simulink model "chapter2"  (R2022a)
settings: Solver=FixedStepAuto  StartTime=0.0  StopTime=1  FixedStep=1e-3  RelTol=1e-3
model workspace (MAT data in the model file):
  a = 0
values from neighbouring files (symbols this model uses):
  A = 10    [Figure2_3.m]    (also in Figure2_9and2_10and2_11.m = A_set(N1-5); parameterLoadForchapter2_4.m = 0.0001; parameterLoadForchapter2_5.m = 0.0001; parameter_load3.m = 0.01)
  Ln = Lns(i)    [Figure2_12and2_13.m]    (also in Figure2_14and2_15.m; Figure2_16and2_17.m; Mchapter2_4.m = LNs(i); parameterLoadForchapter2_5.m = 0.02)
  r = 0.42    [parameterLoadForchapter2_4.m]    (also in parameterLoadForchapter2_5.m; parameter_load3.m)
  v = 100/3.6    (= 27.7777777778)    [Figure2_18_and2_19.m]    (also in Figure2_20_and2_21.m; parameterLoadForchapter2_4.m = 13.8888888889; parameterLoadForchapter2_5.m; parameter_load3.m)
undefined symbols (not defined in the file or in its folder): C1, K1, M1
settings Model: Creator=Spicydel  LastModifiedBy=Spicydel

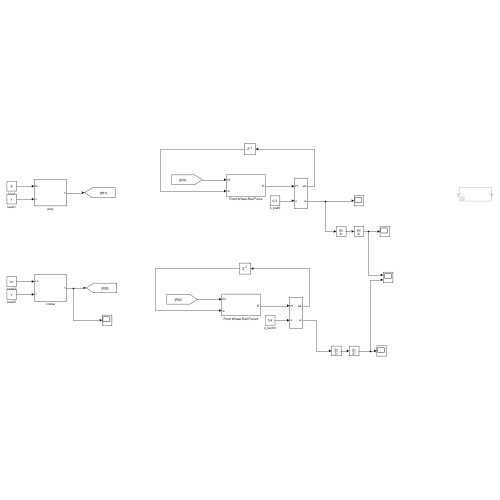
[thumbnail: Simulink's stored preview of the top-level diagram]
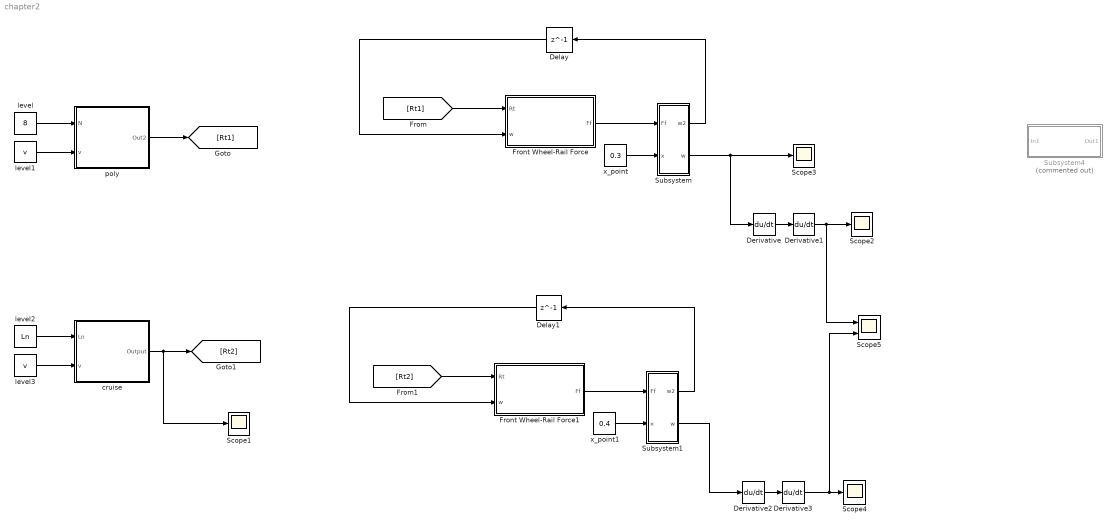
== system chapter2 ==
  Delay : Delay  DelayLength=1
  Delay1 : Delay  DelayLength=1
  Derivative{,1..3} (4 alike) : Derivative
  Front Wheel-Rail Force : Subsystem
  Front Wheel-Rail Force1 : Subsystem
  Scope{1..4} (4 alike) : Scope
  Scope5 : Scope  NumInputPorts=2
  Subsystem : Subsystem
  Subsystem1 : Subsystem
  Subsystem4 : Subsystem  Commented=on
  cruise : Subsystem
  level : Constant  Value=8
  level1 : Constant  Value=v
  level2 : Constant  Value=Ln
  level3 : Constant  Value=v
  poly : Subsystem
  x_point : Constant  Value=0.3
  x_point1 : Constant  Value=0.4
  wires:
  Front Wheel-Rail Force/1(Ff) -> Subsystem/1(Ff)
  x_point/1 -> Subsystem/2(x)
  Derivative/1 -> Derivative1/1
  Delay/1 -> Front Wheel-Rail Force/2(w)
  level/1 -> poly/1(N)
  level1/1 -> poly/2(v)
  poly/1(Out2) -> [Rt1]
  [Rt1] -> Front Wheel-Rail Force/1(Rt)
  cruise/1(Output) -> Scope1/1, [Rt2]
  level3/1 -> cruise/2(v)
  level2/1 -> cruise/1(Ln)
  [Rt2] -> Front Wheel-Rail Force1/1(Rt)
  Delay1/1 -> Front Wheel-Rail Force1/2(w)
  Derivative2/1 -> Derivative3/1
  x_point1/1 -> Subsystem1/2(x)
  Front Wheel-Rail Force1/1(Ff) -> Subsystem1/1(Ff)
  Derivative1/1 -> Scope5/1, Scope2/1
  Derivative3/1 -> Scope5/2, Scope4/1
  Subsystem/1(w2) -> Delay/1
  Subsystem/2(w) -> Derivative/1, Scope3/1
  Subsystem1/1(w2) -> Delay1/1
  Subsystem1/2(w) -> Derivative2/1

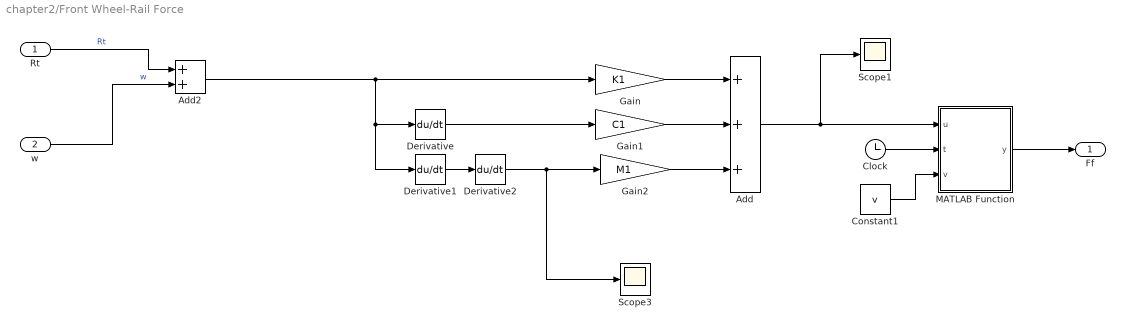
== system chapter2/Front Wheel-Rail Force ==
  Rt : Inport
  w : Inport  Port=2
  Add : Sum  Inputs=+++
  Add2 : Sum
  Clock : Clock
  Constant1 : Constant  Value=v
  Derivative : Derivative
  Derivative1 : Derivative
  Derivative2 : Derivative
  Gain : Gain  Gain=K1
  Gain1 : Gain  Gain=C1
  Gain2 : Gain  Gain=M1
  MATLAB Function : MATLAB Function  TreatAsAtomicUnit=on
  Scope1 : Scope
  Scope3 : Scope
  Ff : Outport
  wires:
  Add2/1 -> Gain/1, Derivative1/1, Derivative/1
  Derivative1/1 -> Derivative2/1
  Gain2/1 -> Add/3
  Gain/1 -> Add/1
  Add/1 -> Scope1/1, MATLAB Function/1(u)
  Rt/1 -> Add2/1  "Rt"
  w/1 -> Add2/2  "w"
  MATLAB Function/1(y) -> Ff/1
  Clock/1 -> MATLAB Function/2(t)
  Constant1/1 -> MATLAB Function/3(v)
  Derivative2/1 -> Scope3/1, Gain2/1
  Derivative/1 -> Gain1/1
  Gain1/1 -> Add/2

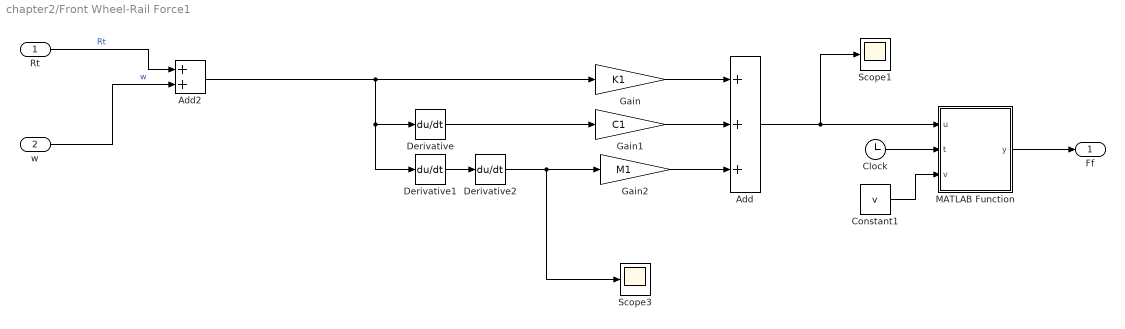
== system chapter2/Front Wheel-Rail Force1 ==
  Rt : Inport
  w : Inport  Port=2
  Add : Sum  Inputs=+++
  Add2 : Sum
  Clock : Clock
  Constant1 : Constant  Value=v
  Derivative : Derivative
  Derivative1 : Derivative
  Derivative2 : Derivative
  Gain : Gain  Gain=K1
  Gain1 : Gain  Gain=C1
  Gain2 : Gain  Gain=M1
  MATLAB Function : MATLAB Function  TreatAsAtomicUnit=on
  Scope1 : Scope
  Scope3 : Scope
  Ff : Outport
  wires:
  Gain1/1 -> Add/2
  Derivative/1 -> Gain1/1
  Derivative2/1 -> Gain2/1, Scope3/1
  Constant1/1 -> MATLAB Function/3(v)
  Clock/1 -> MATLAB Function/2(t)
  MATLAB Function/1(y) -> Ff/1
  w/1 -> Add2/2  "w"
  Rt/1 -> Add2/1  "Rt"
  Add/1 -> MATLAB Function/1(u), Scope1/1
  Gain/1 -> Add/1
  Gain2/1 -> Add/3
  Derivative1/1 -> Derivative2/1
  Add2/1 -> Derivative/1, Derivative1/1, Gain/1

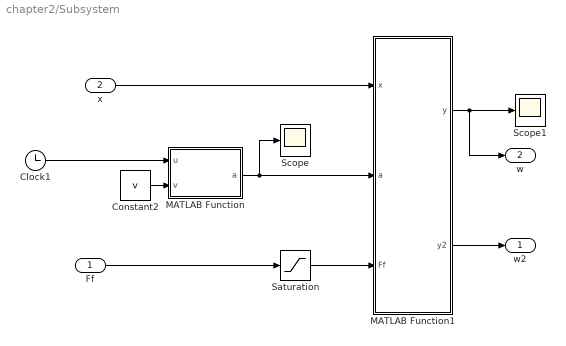
== system chapter2/Subsystem ==
  Ff : Inport
  x : Inport  Port=2
  Clock1 : Clock
  Constant2 : Constant  Value=v
  MATLAB Function : MATLAB Function  TreatAsAtomicUnit=on
  MATLAB Function1 : MATLAB Function  TreatAsAtomicUnit=on
  Saturation : Saturate  UpperLimit=1.5*100000  LowerLimit=0
  Scope : Scope
  Scope1 : Scope
  w2 : Outport
  w : Outport  Port=2
  wires:
  Ff/1 -> Saturation/1
  MATLAB Function/1(a) -> Scope/1, MATLAB Function1/2(a)
  Clock1/1 -> MATLAB Function/1(u)
  Constant2/1 -> MATLAB Function/2(v)
  x/1 -> MATLAB Function1/1(x)
  Saturation/1 -> MATLAB Function1/3(Ff)
  MATLAB Function1/1(y) -> w/1, Scope1/1
  MATLAB Function1/2(y2) -> w2/1

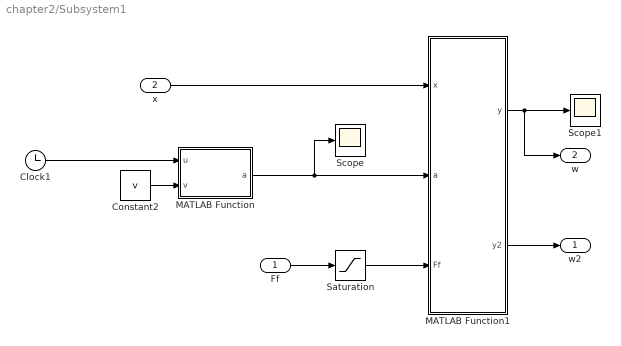
== system chapter2/Subsystem1 ==
  Ff : Inport
  x : Inport  Port=2
  Clock1 : Clock
  Constant2 : Constant  Value=v
  MATLAB Function : MATLAB Function  TreatAsAtomicUnit=on
  MATLAB Function1 : MATLAB Function  TreatAsAtomicUnit=on
  Saturation : Saturate  UpperLimit=1.5*100000  LowerLimit=0
  Scope : Scope
  Scope1 : Scope
  w2 : Outport
  w : Outport  Port=2
  wires:
  Ff/1 -> Saturation/1
  MATLAB Function/1(a) -> Scope/1, MATLAB Function1/2(a)
  Clock1/1 -> MATLAB Function/1(u)
  Constant2/1 -> MATLAB Function/2(v)
  x/1 -> MATLAB Function1/1(x)
  Saturation/1 -> MATLAB Function1/3(Ff)
  MATLAB Function1/1(y) -> w/1, Scope1/1
  MATLAB Function1/2(y2) -> w2/1

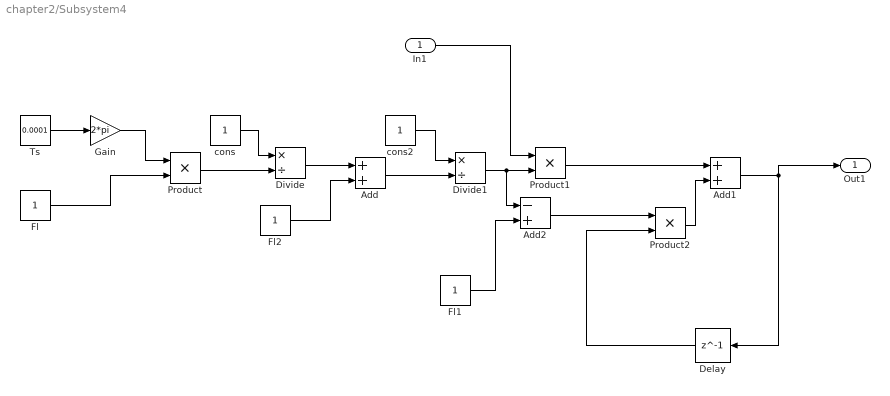
== system chapter2/Subsystem4 ==
  In1 : Inport
  Add : Sum
  Add1 : Sum
  Add2 : Sum  Inputs=-+
  Delay : Delay  DelayLength=1
  Divide : Product  Inputs=*/
  Divide1 : Product  Inputs=*/
  Fl : Constant
  Fl1 : Constant
  Fl2 : Constant
  Gain : Gain  Gain=2*pi
  Product : Product
  Product1 : Product
  Product2 : Product
  Ts : Constant  Value=0.0001
  cons : Constant
  cons2 : Constant
  Out1 : Outport
  wires:
  Ts/1 -> Gain/1
  Fl/1 -> Product/2
  Gain/1 -> Product/1
  Product/1 -> Divide/2
  cons/1 -> Divide/1
  Divide/1 -> Add/1
  Fl2/1 -> Add/2
  Add/1 -> Divide1/2
  cons2/1 -> Divide1/1
  Divide1/1 -> Add2/1, Product1/2
  In1/1 -> Product1/1
  Add1/1 -> Delay/1, Out1/1
  Delay/1 -> Product2/2
  Product2/1 -> Add1/2
  Product1/1 -> Add1/1
  Fl1/1 -> Add2/2
  Add2/1 -> Product2/1

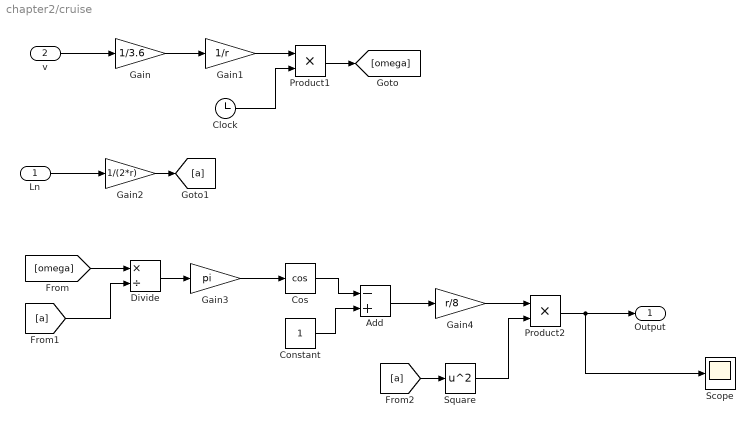
== system chapter2/cruise ==
  Ln : Inport
  v : Inport  Port=2
  Add : Sum  Inputs=-+
  Clock : Clock
  Constant : Constant
  Cos : Trigonometry  Operator=cos
  Divide : Product  Inputs=*/
  Gain : Gain  Gain=1/3.6
  Gain1 : Gain  Gain=1/r
  Gain2 : Gain  Gain=1/(2*r)
  Gain3 : Gain  Gain=pi
  Gain4 : Gain  Gain=r/8
  Product1 : Product
  Product2 : Product
  Scope : Scope
  Square : Math  Operator=square
  Output : Outport
  wires:
  Product1/1 -> [omega]
  Clock/1 -> Product1/2
  Gain1/1 -> Product1/1
  Gain/1 -> Gain1/1
  v/1 -> Gain/1
  Ln/1 -> Gain2/1
  Gain2/1 -> [a]
  [omega] -> Divide/1
  [a] -> Divide/2
  Divide/1 -> Gain3/1
  Gain3/1 -> Cos/1
  Constant/1 -> Add/2
  Cos/1 -> Add/1
  Add/1 -> Gain4/1
  Gain4/1 -> Product2/1
  [a] -> Square/1
  Square/1 -> Product2/2
  Product2/1 -> Output/1, Scope/1

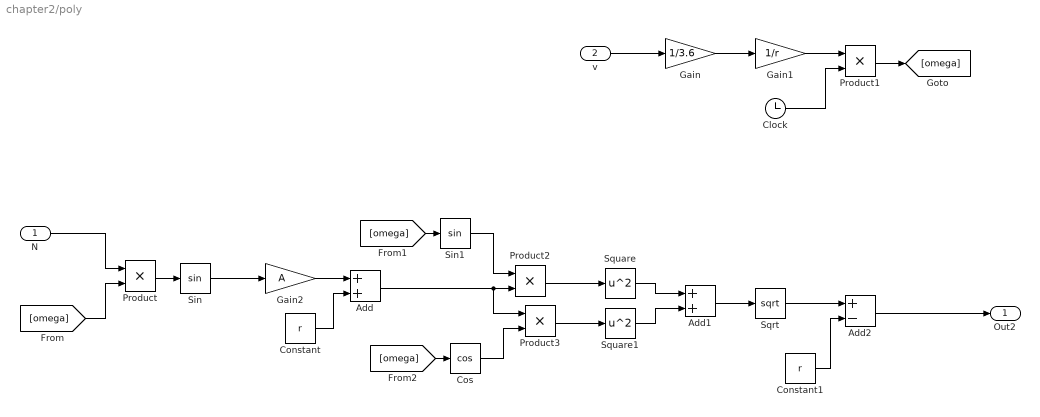
== system chapter2/poly ==
  N : Inport
  v : Inport  Port=2
  Add : Sum
  Add1 : Sum
  Add2 : Sum  Inputs=+-
  Clock : Clock
  Constant : Constant  Value=r
  Constant1 : Constant  Value=r
  Cos : Trigonometry  Operator=cos
  Gain : Gain  Gain=1/3.6
  Gain1 : Gain  Gain=1/r
  Gain2 : Gain  Gain=A
  Product{,1..3} (4 alike) : Product
  Sin : Trigonometry
  Sin1 : Trigonometry
  Sqrt : Sqrt
  Square : Math  Operator=square
  Square1 : Math  Operator=square
  Out2 : Outport
  wires:
  v/1 -> Gain/1
  Gain/1 -> Gain1/1
  N/1 -> Product/1
  Gain1/1 -> Product1/1
  Clock/1 -> Product1/2
  Product1/1 -> [omega]
  [omega] -> Product/2
  Product/1 -> Sin/1
  Sin/1 -> Gain2/1
  Gain2/1 -> Add/1
  Constant/1 -> Add/2
  [omega] -> Sin1/1
  Add/1 -> Product3/1, Product2/2
  Sin1/1 -> Product2/1
  Cos/1 -> Product3/2
  [omega] -> Cos/1
  Square1/1 -> Add1/2
  Product2/1 -> Square/1
  Square/1 -> Add1/1
  Sqrt/1 -> Add2/1
  Add1/1 -> Sqrt/1
  Product3/1 -> Square1/1
  Constant1/1 -> Add2/2
  Add2/1 -> Out2/1

== matlab function chapter2/Front Wheel-Rail Force/MATLAB Function ==
  data: u input; y output; t input; v input
function y = fcn(u, t , v)
t0 = 0.5;
t1 = 0.6/(v/3.6);
t2 = 2.6/(v/3.6);
M1 = 1723*9.8;
M = (32988+4060)*9.8;
if t <= (t1+t0) &&t >= t0
    y = u + M1 + M/4;
elseif t > (t2 + t0) && t <= (t0 + t1 + t2)
    y = u + M1 + M/4;
else
    y = 0;
end

end

== matlab function chapter2/Subsystem/MATLAB Function ==
  data: u input; a output; v input
function a = fcn(u,v)
t0 = 0.5;
t1 = t0 + 0.6/(v/3.6);
t2 = t0 + 2.6/(v/3.6);
    if u <= t1 && u >t0
        a = (u-t0)*v/3.6;
    elseif u > t2 && u <= (t1 + t2 -t0)
        a = (u-t2)*v/3.6;
    else
        a = 0;
    end
end

== matlab function chapter2/Subsystem1/MATLAB Function ==
  data: u input; a output; v input
function a = fcn(u,v)
t0 = 0.5;
t1 = t0 + 0.6/(v/3.6);
t2 = t0 + 2.6/(v/3.6);
    if u <= t1 && u >t0
        a = (u-t0)*v/3.6;
    elseif u > t2 && u <= (t1 + t2 -t0)
        a = (u-t2)*v/3.6;
    else
        a = 0;
    end
end

== matlab function chapter2/Subsystem1/MATLAB Function1 ==
  data: x input; y output; a input; Ff input; y2 output
function [y,y2] = fcn(x,a, Ff)
l = 0.6
b = l - a;
E = 2*10^11;
I = 4.489 * 10^(-5);

if x <= a
    y = Ff*b*x*(l*l-x*x-b*b)/6/l/E/I;
else
    y = Ff*a*(l-x)*(2*l*x-x*x-a*a)/6/l/E/I;
end

y2 = Ff*a*b*(l*l-a*a-b*b)/6/l/E/I;
end

== matlab function chapter2/Front Wheel-Rail Force1/MATLAB Function ==
  data: u input; y output; t input; v input
function y = fcn(u, t , v)
t0 = 0.5;
t1 = 0.6/(v/3.6);
t2 = 2.6/(v/3.6);
M1 = 1723*9.8;
M = (32988+4060)*9.8;
if t <= (t1+t0) &&t >= t0
    y = u + M1 + M/4;
elseif t > (t2 + t0) && t <= (t0 + t1 + t2)
    y = u + M1 + M/4;
else
    y = 0;
end

end

== matlab function chapter2/Subsystem/MATLAB Function1 ==
  data: x input; y output; a input; Ff input; y2 output
function [y,y2] = fcn(x,a, Ff)
l = 0.6
b = l - a;
E = 2*10^11;
I = 4.489 * 10^(-5);

if x <= a
    y = Ff*b*x*(l*l-x*x-b*b)/6/l/E/I;
else
    y = Ff*a*(l-x)*(2*l*x-x*x-a*a)/6/l/E/I;
end

y2 = Ff*a*b*(l*l-a*a-b*b)/6/l/E/I;
end
